simulink subsystem "ElectricalSystemSSC"  (R2025b)
settings: Solver=VariableStepAuto  StartTime=0.0  StopTime=10.0  RelTol=1e-3
undefined symbols (not defined in the file): PlntDCDCVoltInit, ThrmBatt, ThrmEM, ThrmPwrE
libraries: nesl_utility_internal x1
settings Model: ModifiedByFormat=The MathWorks, Inc.  Creator=The MathWorks, Inc.  LastModifiedBy=The MathWorks, Inc.
settings RTWCC: GPUComputeCapability=3.5

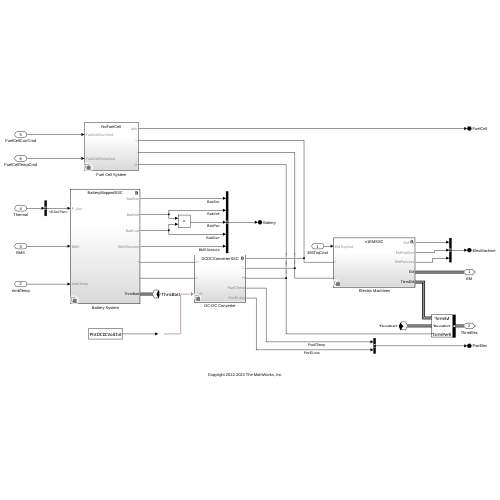
[thumbnail: Simulink's stored preview of the top-level diagram]
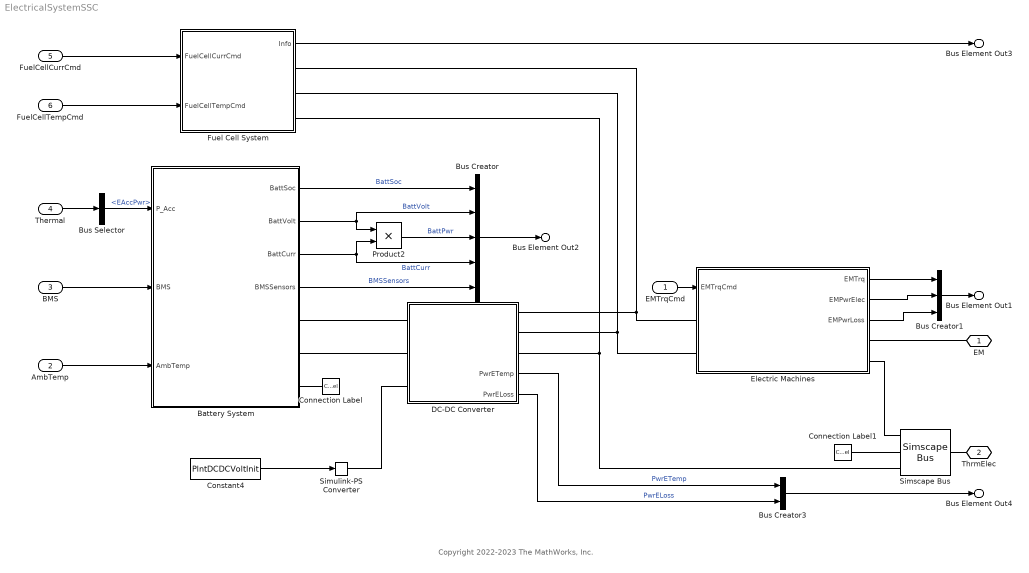
== system ElectricalSystemSSC ==
  note: Copyright 2022-2023 The MathWorks, Inc.
  EMTrqCmd : Inport
  AmbTemp : Inport  Port=2
  BMS : Inport  Port=3
  Thermal : Inport  Port=4
  FuelCellCurrCmd : Inport  Port=5
  FuelCellTempCmd : Inport  Port=6
  Battery System : Subsystem  Variant=on  VariantChoicesSpecifier={'BatteryMappedSSC', 'DetailedBatteryModel'}  VariantControlMode=label  LabelModeActiveChoice=BatteryMappedSSC
  Bus Creator : BusCreator  Inputs=5
  Bus Creator1 : BusCreator  Inputs=3
  Bus Creator3 : BusCreator  Inputs=2
  Bus Selector : BusSelector  OutputSignals=EAccPwr
  Connection Label : ConnectionLabel  Label=ThrmBatt
  Connection Label1 : ConnectionLabel  Label=ThrmBatt
  Constant4 : Constant  Value=PlntDCDCVoltInit  SampleTime=-1
  DC-DC Converter : Subsystem  Variant=on  VariantChoicesSpecifier={'DCDCConverterSSC', 'NoDCDCConverterSSC'}  VariantControlMode=label  VariantControl=Choice  LabelModeActiveChoice=DCDCConverterSSC
      settings: PortSchema="{\"entries\":[{\"content\":{\"sides\":[{\"content\":{\"connectorIds\":[\"LConn1\",\"LConn2\",\"LConn3\"]},\"type\":\"ConnectorPlacement.EquallySpacedRectSide\",\"uuid\":\"52670659-127e-44f2-81d3-442cf6c9e083\"},{\"content\":{\"connectorIds\":[\"RConn1\",\"RConn2\",\"RConn3\",\"Out1\",\"Out2\"],\"side\":\"RIGHT\"},\"type\":\"ConnectorPlacement.EquallySpacedRectSide\",\"uuid\":\"5896ffba-a38c-48c1-a001-3097ae388e27\"},{\"content\":{\"side\":\"TOP\"},\"type\":\"ConnectorPlacement.EquallySpacedRectSide\",\"uuid\":\"e63e50d5-c739-4c67-ba83-2c3ff28a87dd\"}]},\"type\":\"ConnectorPlacement.EquallySpacedConnector\",\"uuid\":\"70f69b26-fc9f-4b50-9575-916c48862b31\"}],\"packageUris\":[\"http://schema.mathworks.com/mf0/Connector/R2020b\"],\"version\":\"1.0\"}"
  Electric Machines : Subsystem  Variant=on  VariantChoicesSpecifier={'s1EMSSC', 's2EMSSC', 's3EMSSC', 's4EMSSC'}  VariantControlMode=label  VariantControl=Choice  LabelModeActiveChoice=s1EMSSC
  Fuel Cell System : Subsystem  Variant=on  VariantControlMode=label  LabelModeActiveChoice=NoFuelCell
  Product2 : Product
  Simscape Bus : SimscapeBus  HierarchyStrings=ThrmEM;ThrmBatt;ThrmPwrE
  Simulink-PS Converter : nesl_utility_internal/Simulink-PS Converter  PhysicalDomain=network_engine_domain  SubClassName=ps_input  LeftPortType=input  RightPortType=output  PseudoPeriodic=off  Frequencies=[]  NoiseDistribution=none  NoiseParameters=[]  Unit=1  AffineConversion=off  FilteringAndDerivatives=provide  SimscapeFilterOrder=1  InputFilterTimeConstant=0.001  UdotUserProvided=0
  EM : PMIOPort  Side=Right
  ThrmElec : PMIOPort  Port=2  Side=Right
  Bus Element Out2 : Outport  PortName=Battery
  Bus Element Out1 : Outport  Port=2  PortName=ElecMachine
  Bus Element Out3 : Outport  Port=3  PortName=FuelCell
  Bus Element Out4 : Outport  Port=4  PortName=PwrElec
  wires:
  Electric Machines/2(EMPwrElec) -> Bus Creator1/2
  Electric Machines/1(EMTrq) -> Bus Creator1/1
  EMTrqCmd/1 -> Electric Machines/1(EMTrqCmd)
  Battery System/4(BMSSensors) -> Bus Creator/5  "BMSSensors"
  AmbTemp/1 -> Battery System/3(AmbTemp)
  BMS/1 -> Battery System/2(BMS)
  Constant4/1 -> Simulink-PS Converter/1
  Product2/1 -> Bus Creator/3  "BattPwr"
  Battery System/1(BattSoc) -> Bus Creator/1  "BattSoc"
  Battery System/3(BattCurr) -> Bus Creator/4, Product2/2  "BattCurr"
  Battery System/2(BattVolt) -> Product2/1, Bus Creator/2  "BattVolt"
  Bus Creator/1 -> Bus Element Out2/1
  Bus Creator1/1 -> Bus Element Out1/1
  Bus Selector/1 -> Battery System/1(P_Acc)  "<EAccPwr>"
  Thermal/1 -> Bus Selector/1
  FuelCellCurrCmd/1 -> Fuel Cell System/1(FuelCellCurrCmd)
  Fuel Cell System/1(Info) -> Bus Element Out3/1
  FuelCellTempCmd/1 -> Fuel Cell System/2(FuelCellTempCmd)
  Electric Machines/3(EMPwrLoss) -> Bus Creator1/3
  Bus Creator3/1 -> Bus Element Out4/1
  DC-DC Converter/1(PwrETemp) -> Bus Creator3/1  "PwrETemp"
  DC-DC Converter/2(PwrELoss) -> Bus Creator3/2  "PwrELoss"
  connections:
  Electric Machines/LConn2 -- Fuel Cell System/RConn2 -- DC-DC Converter/RConn2
  Electric Machines/LConn1 -- Fuel Cell System/RConn1 -- DC-DC Converter/RConn1
  DC-DC Converter/RConn3 -- Simscape Bus/LConn3 -- Fuel Cell System/RConn3
  Electric Machines/RConn1 -- EM/RConn1
  Battery System/RConn2 -- DC-DC Converter/LConn2
  Battery System/RConn1 -- DC-DC Converter/LConn1
  Simulink-PS Converter/RConn1 -- DC-DC Converter/LConn3
  Simscape Bus/RConn1 -- ThrmElec/RConn1
  Connection Label/LConn1 -- Battery System/RConn3
  Connection Label1/LConn1 -- Simscape Bus/LConn2
  Simscape Bus/LConn1 -- Electric Machines/RConn2

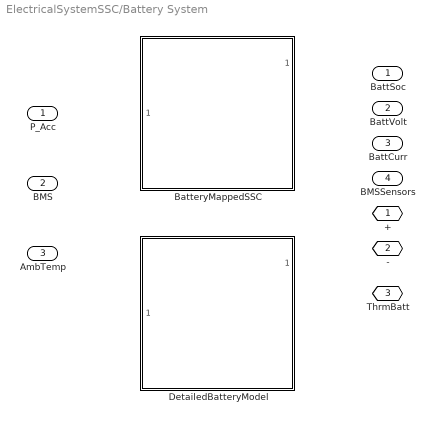
== system ElectricalSystemSSC/Battery System ==
  P_Acc : Inport
  BMS : Inport  Port=2
  AmbTemp : Inport  Port=3
  BatteryMappedSSC : Subsystem  VariantControl=BatteryMappedSSC  ReferencedSubsystem=BatteryMappedSSC
  DetailedBatteryModel : Subsystem  VariantControl=DetailedBatteryModel  ReferencedSubsystem=DetailedBatteryModel
  + : PMIOPort  Side=Right
  - : PMIOPort  Port=2  Side=Right
  ThrmBatt : PMIOPort  Port=3  Side=Right
  BattSoc : Outport  VectorParamsAs1DForOutWhenUnconnected=off
  BattVolt : Outport  Port=2  VectorParamsAs1DForOutWhenUnconnected=off
  BattCurr : Outport  Port=3  VectorParamsAs1DForOutWhenUnconnected=off
  BMSSensors : Outport  Port=4  VectorParamsAs1DForOutWhenUnconnected=off

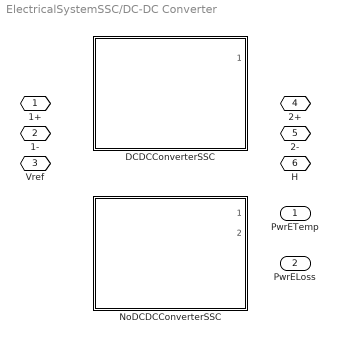
== system ElectricalSystemSSC/DC-DC Converter ==
  DCDCConverterSSC : Subsystem  VariantControl=DCDCConverterSSC  ReferencedSubsystem=DCDCConverterSSC
  NoDCDCConverterSSC : Subsystem  VariantControl=NoDCDCConverterSSC  ReferencedSubsystem=NoDCDCConverterSSC
  1+ : PMIOPort  Side=Left
  1- : PMIOPort  Port=2  Side=Left
  Vref : PMIOPort  Port=3  Side=Left
  2+ : PMIOPort  Port=4  Side=Right
  2- : PMIOPort  Port=5  Side=Right
  H : PMIOPort  Port=6  Side=Right
  PwrETemp : Outport
  PwrELoss : Outport  Port=2

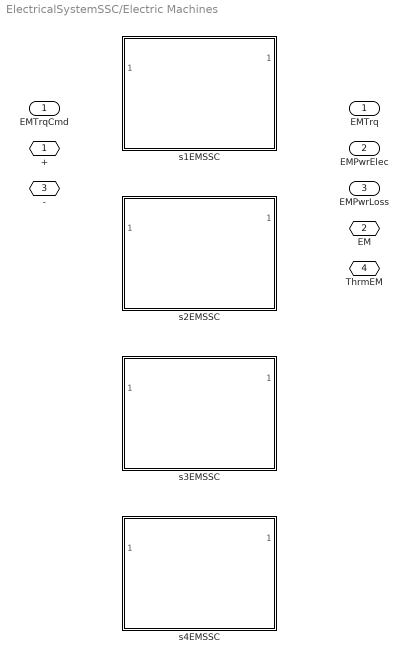
== system ElectricalSystemSSC/Electric Machines ==
  EMTrqCmd : Inport
  s1EMSSC : Subsystem  VariantControl=s1EMSSC  ReferencedSubsystem=s1EMSSC
  s2EMSSC : Subsystem  VariantControl=s2EMSSC  ReferencedSubsystem=s2EMSSC
  s3EMSSC : Subsystem  VariantControl=s3EMSSC  ReferencedSubsystem=s3EMSSC
  s4EMSSC : Subsystem  VariantControl=s4EMSSC  ReferencedSubsystem=s4EMSSC
  + : PMIOPort  Side=Left
  EM : PMIOPort  Port=2  Side=Right
  - : PMIOPort  Port=3  Side=Left
  ThrmEM : PMIOPort  Port=4  Side=Right
  EMTrq : Outport
  EMPwrElec : Outport  Port=2
  EMPwrLoss : Outport  Port=3

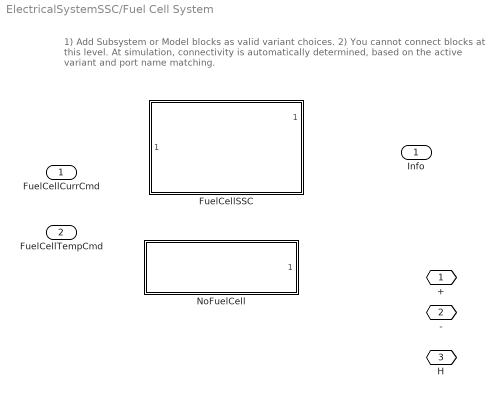
== system ElectricalSystemSSC/Fuel Cell System ==
  note: 1) Add Subsystem or Model blocks as valid variant choices.
      | 2) You cannot connect blocks at this level. At simulation, connectivity is automatically
      | determined, based on the active variant and port name matching.
  FuelCellCurrCmd : Inport
  FuelCellTempCmd : Inport  Port=2
  FuelCellSSC : Subsystem  VariantControl=FuelCellSSC  ReferencedSubsystem=FuelCellSSC
  NoFuelCell : Subsystem  VariantControl=NoFuelCell  ReferencedSubsystem=NoFuelCell
  + : PMIOPort  Side=Right
  - : PMIOPort  Port=2  Side=Right
  H : PMIOPort  Port=3  Side=Right
  Info : Outport
